simulink model "Hw4_ME8352sim"  (R2020b)
settings: Solver=VariableStepAuto  StartTime=0.0  StopTime=t_sim  RelTol=1e-5
values from neighbouring files (symbols this model uses):
  F0 = 1    [Hw4_ME8352.m]
  k_ = 1    [Hw4_ME8352.m]
  m = 1    [Hw4_ME8352.m]
  x_0 = x0_array(ii)    [Hw4_ME8352.m]
  xdot_0 = xdot0_array(iii)    [Hw4_ME8352.m]
settings Model: Creator=dempseca  LastModifiedBy=dempseca
settings DebuggingCC: IgnoredZcDiagnostic=none

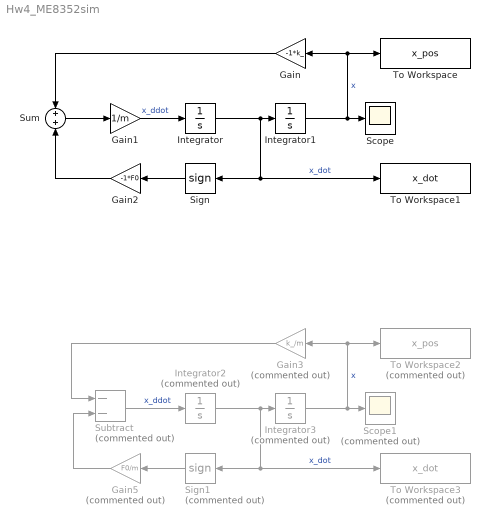
== system Hw4_ME8352sim ==
  Gain : Gain  Gain=-1*k_
  Gain1 : Gain  Gain=1/m
  Gain2 : Gain  Gain=-1*F0
  Gain3 : Gain  Commented=on  Gain=k_/m
  Gain5 : Gain  Commented=on  Gain=F0/m
  Integrator : Integrator  InitialCondition=xdot_0  LimitOutput=on  UpperSaturationLimit=100  LowerSaturationLimit=-100
  Integrator1 : Integrator  InitialCondition=x_0  LimitOutput=on  UpperSaturationLimit=100  LowerSaturationLimit=-100
  Integrator2 : Integrator  Commented=on  InitialCondition=xdot_0  UpperSaturationLimit=100
  Integrator3 : Integrator  Commented=on  InitialCondition=x_0  UpperSaturationLimit=100  LowerSaturationLimit=-100
  Scope : Scope
  Scope1 : Scope  Commented=on
  Sign : Signum  ZeroCross=off
  Sign1 : Signum  Commented=on  ZeroCross=off
  Subtract : Sum  Commented=on  Inputs=--
  Sum : Sum
  To Workspace : ToWorkspace  VariableName=x_pos  SaveFormat=Timeseries  SampleTime=-1
  To Workspace1 : ToWorkspace  VariableName=x_dot  SaveFormat=Timeseries  SampleTime=-1
  To Workspace2 : ToWorkspace  Commented=on  VariableName=x_pos  SaveFormat=Timeseries  SampleTime=-1
  To Workspace3 : ToWorkspace  Commented=on  VariableName=x_dot  SaveFormat=Timeseries  SampleTime=-1
  wires:
  Integrator/1 -> To Workspace1/1, Sign/1, Integrator1/1  "x_dot"
  Integrator1/1 -> To Workspace/1, Gain/1, Scope/1  "x"
  Sum/1 -> Gain1/1
  Gain/1 -> Sum/1
  Gain1/1 -> Integrator/1  "x_ddot"
  Sign/1 -> Gain2/1
  Gain2/1 -> Sum/2
  Sign1/1 -> Gain5/1
  Gain3/1 -> Subtract/1
  Integrator2/1 -> To Workspace3/1, Sign1/1, Integrator3/1  "x_dot"
  Gain5/1 -> Subtract/2
  Integrator3/1 -> To Workspace2/1, Gain3/1, Scope1/1  "x"
  Subtract/1 -> Integrator2/1  "x_ddot"
